simulink model "mat_model"  (R2023a)
settings: Solver=ode4  StartTime=0  StopTime=0.3  FixedStep=1e-7  RelTol=1e-3  EnableMultiTasking=on
undefined symbols (not defined in the file): a_noise, adc_delay_length, ADC_max, adc_sample, b_noise, borehole_max, C_e, C_m, clock_for_random, degrees_shaft_max, delay_ADC, delay_calc_borehole, J_en, J_load, K_degrees2borehole, K_integral, K_noise, K_potentiometer, K_proportional, offset_potentiometer, phi_demanded, q, q_stage, R_rotor, STEP_INTEGRAL, T_rotor, theta_max, U_en_supply, U_ref, width_window
libraries: eePwmGenerator x1
settings Model: SimulationMode=accelerator  Creator=Admin  LastModifiedBy=Director
settings SolverCC: NumberNewtonIterations=4  AlgebraicLoopSolver=TrustRegion  AutoInsertRateTranBlk=on
settings DataIOCC: LimitDataPoints=on  SaveFormat=Array  SignalLoggingSaveFormat=ModelDataLogs  SaveOutput=off  ReturnWorkspaceOutputs=off
settings OptimizationCC: ExpressionDepthLimit=2147483647  LifeSpan=inf  SimCompilerOptimization=on
settings DebuggingCC: UnderspecifiedInitializationDetection=Classic  MergeDetectMultiDrivingBlocksExec=none  SolverPrmCheckMsg=warning  FcnCallInpInsideContextMsg=warning  UnconnectedInputMsg=warning  UnconnectedOutputMsg=warning  UnconnectedLineMsg=warning  StateNameClashWarn=warning  SFUnexpectedBacktrackingDiag=warning  SFNoUnconditionalDefaultTransitionDiag=warning  SFExecutionAtInitializationDiag=none  ArithmeticOperatorsInVariantConditions=warning
settings HardwareCC: ProdBitPerLong=64  ProdLargestAtomicFloat=None  ProdHWDeviceType=AMD->Athlon 64
settings ModelReferenceCC: EnableRefExpFcnMdlSchedulingChecks=on  PropagateSignalLabelsOutOfModel=off
settings SFSimCC: SimUseLocalCustomCode=off  CustomCodeUndefinedFunction=UseInterfaceOnly
settings RTWCC: RTWUseLocalCustomCode=off
settings CodeAppCC: StateflowObjectComments=on
settings GRTTargetCC: TargetLangStandard=C89/C90 (ANSI)  CombineOutputUpdateFcns=off  GRTInterface=on
settings ConfigComp: CovMetricSettings=dw  CovSaveCumulativeToWorkspaceVar=on  CovSaveSingleToWorkspaceVar=on  CovExternalEMLEnable=off
settings SimscapeCC: SimscapeNormalizeSystem=off
settings ConfigurationSet: Description=SimMechanics 2G

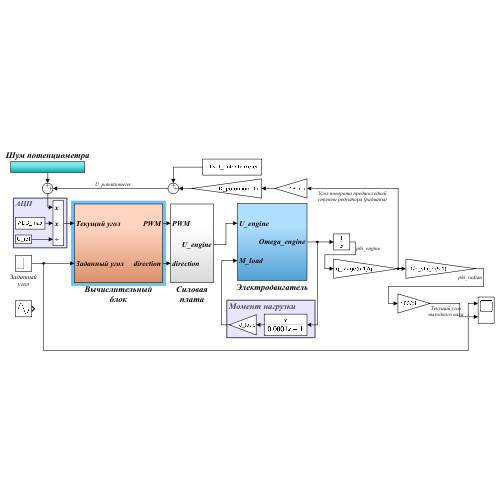
[thumbnail: Simulink's stored preview of the top-level diagram]
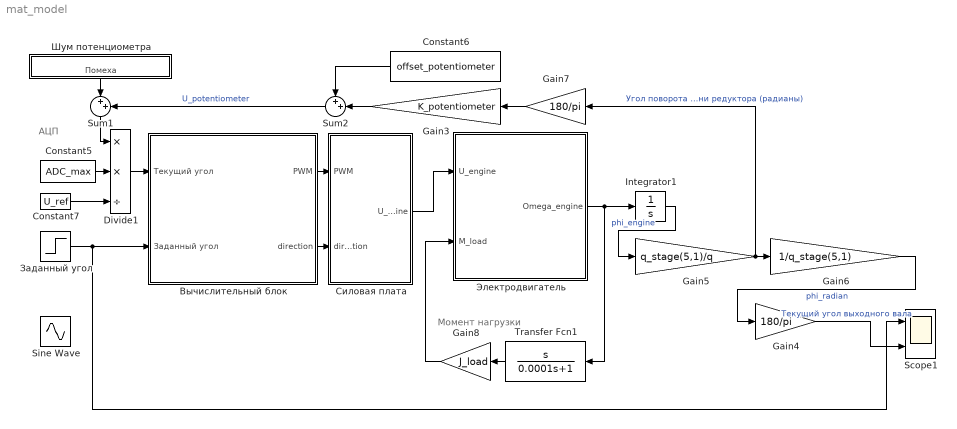
== system mat_model ==
  note: Момент нагрузки
  note: АЦП
  Constant5 : Constant  Value=ADC_max
  Constant6 : Constant  Value=offset_potentiometer
  Constant7 : Constant  Value=U_ref
  Divide1 : Product  Inputs=**/
  Gain3 : Gain  Gain=K_potentiometer
  Gain4 : Gain  Gain=180/pi
  Gain5 : Gain  Gain=q_stage(5,1)/q
  Gain6 : Gain  Gain=1/q_stage(5,1)
  Gain7 : Gain  Gain=180/pi
  Gain8 : Gain  Gain=J_load
  Integrator1 : Integrator
  Scope1 : Scope  NumInputPorts=2
  Sine Wave : Sin  Amplitude=phi_demanded  Frequency=2 * pi * 28.0  SampleTime=0
  Sum1 : Sum  Inputs=|++
  Sum2 : Sum  Inputs=++|
  Transfer Fcn1 : TransferFcn  Numerator=[1 0]  Denominator=[0.0001 1]
  Вычислительный блок : Subsystem
  Заданный угол : Step  Time=0  After=phi_demanded  SampleTime=0
  Силовая плата : Subsystem
  Шум потенциометра : Subsystem
  Электродвигатель : Subsystem
  wires:
  Constant6/1 -> Sum2/1
  Divide1/1 -> Вычислительный блок/1(Текущий угол)
  Gain6/1 -> Gain4/1  "phi_radian"
  Transfer Fcn1/1 -> Gain8/1
  Constant7/1 -> Divide1/3
  Sum1/1 -> Divide1/1
  Gain7/1 -> Gain3/1
  Gain8/1 -> Электродвигатель/2(M_load)
  Integrator1/1 -> Gain5/1  "phi_engine"
  Gain5/1 -> Gain6/1, Gain7/1  "Угол поворота предпоследней ступени редуктора (радианы)"
  Электродвигатель/1(Omega_engine) -> Transfer Fcn1/1, Integrator1/1
  Sum2/1 -> Sum1/2  "U_potentiometer"
  Gain4/1 -> Scope1/2  "Текущий угол выходного вала"
  Constant5/1 -> Divide1/2
  Gain3/1 -> Sum2/2
  Вычислительный блок/1(PWM) -> Силовая плата/1(PWM)
  Вычислительный блок/2(direction) -> Силовая плата/2(direction)
  Силовая плата/1(U_engine) -> Электродвигатель/1(U_engine)
  Заданный угол/1 -> Scope1/1, Вычислительный блок/2(Заданный угол)
  Шум потенциометра/1(Помеха) -> Sum1/1

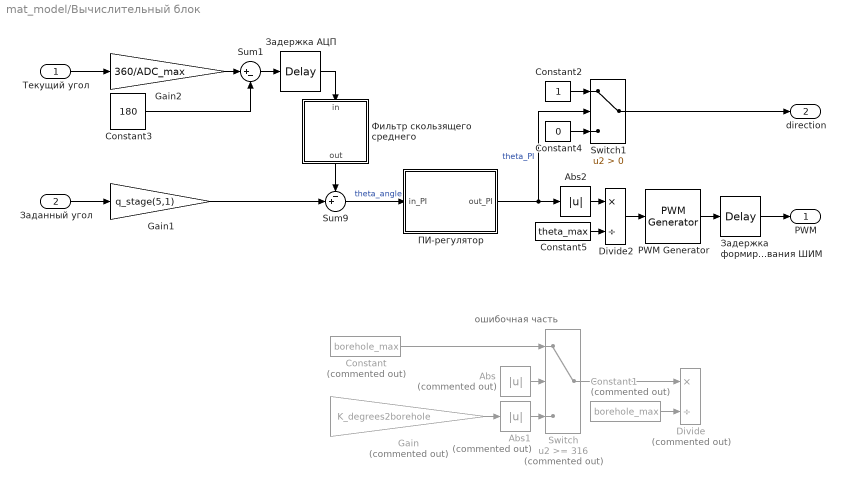
== system mat_model/Вычислительный блок ==
  note: ошибочная часть
  Текущий угол : Inport
  Заданный угол : Inport  Port=2
  Abs : Abs  Commented=on  SaturateOnIntegerOverflow=off
  Abs1 : Abs  Commented=on  SaturateOnIntegerOverflow=off
  Abs2 : Abs  SaturateOnIntegerOverflow=off
  Constant : Constant  Commented=on  Value=borehole_max
  Constant1 : Constant  Commented=on  Value=borehole_max
  Constant2 : Constant
  Constant3 : Constant  Value=180
  Constant4 : Constant  Value=0
  Constant5 : Constant  Value=theta_max
  Divide : Product  Commented=on  Inputs=*/
  Divide2 : Product  Inputs=*/
  Gain : Gain  Commented=on  Gain=K_degrees2borehole
  Gain1 : Gain  Gain=q_stage(5,1)
  Gain2 : Gain  Gain=360/ADC_max
  PWM Generator : eePwmGenerator/PWM Generator  CarrCount=Up  Tper=0.00005  Tdelay=0  Ts=1e-7
  Sum1 : Sum  Inputs=|+-
  Sum9 : Sum  Inputs=-+|
  Switch : Switch  Commented=on  Threshold=316  SaturateOnIntegerOverflow=off  InputSameDT=off
  Switch1 : Switch  Criteria=u2 > Threshold  SaturateOnIntegerOverflow=off  InputSameDT=off
  Задержка формирования ШИМ : TransportDelay  DelayTime=delay_calc_borehole
  Задержка АЦП : TransportDelay  DelayTime=delay_ADC - 0.276*1e-5
  ПИ-регулятор : Subsystem
  Фильтр скользящего среднего : Subsystem
  PWM : Outport
  direction : Outport  Port=2
  wires:
  Sum9/1 -> ПИ-регулятор/1(in_PI)  "theta_angle"
  Задержка формирования ШИМ/1 -> PWM/1
  Constant3/1 -> Sum1/2
  Sum1/1 -> Задержка АЦП/1
  Текущий угол/1 -> Gain2/1
  Gain2/1 -> Sum1/1
  Задержка АЦП/1 -> Фильтр скользящего среднего/1(in)
  Фильтр скользящего среднего/1(out) -> Sum9/1
  Заданный угол/1 -> Gain1/1
  Gain1/1 -> Sum9/2
  Constant/1 -> Switch/1
  Gain/1 -> Abs1/1
  Switch/1 -> Divide/1
  Constant1/1 -> Divide/2
  PWM Generator/1 -> Задержка формирования ШИМ/1
  Constant2/1 -> Switch1/1
  Constant4/1 -> Switch1/3
  Abs/1 -> Switch/2
  Abs1/1 -> Switch/3
  Switch1/1 -> direction/1
  ПИ-регулятор/1(out_PI) -> Switch1/2, Abs2/1  "theta_PI"
  Abs2/1 -> Divide2/1
  Constant5/1 -> Divide2/2
  Divide2/1 -> PWM Generator/1

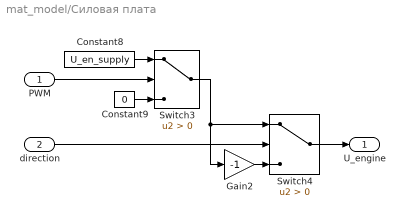
== system mat_model/Силовая плата ==
  PWM : Inport
  direction : Inport  Port=2
  Constant8 : Constant  Value=U_en_supply
  Constant9 : Constant  Value=0
  Gain2 : Gain  Gain=-1
  Switch3 : Switch  Criteria=u2 > Threshold  SaturateOnIntegerOverflow=off  InputSameDT=off
  Switch4 : Switch  Criteria=u2 > Threshold  SaturateOnIntegerOverflow=off  InputSameDT=off
  U_engine : Outport
  wires:
  Constant9/1 -> Switch3/3
  PWM/1 -> Switch3/2
  Switch4/1 -> U_engine/1
  Constant8/1 -> Switch3/1
  direction/1 -> Switch4/2
  Gain2/1 -> Switch4/3
  Switch3/1 -> Switch4/1, Gain2/1

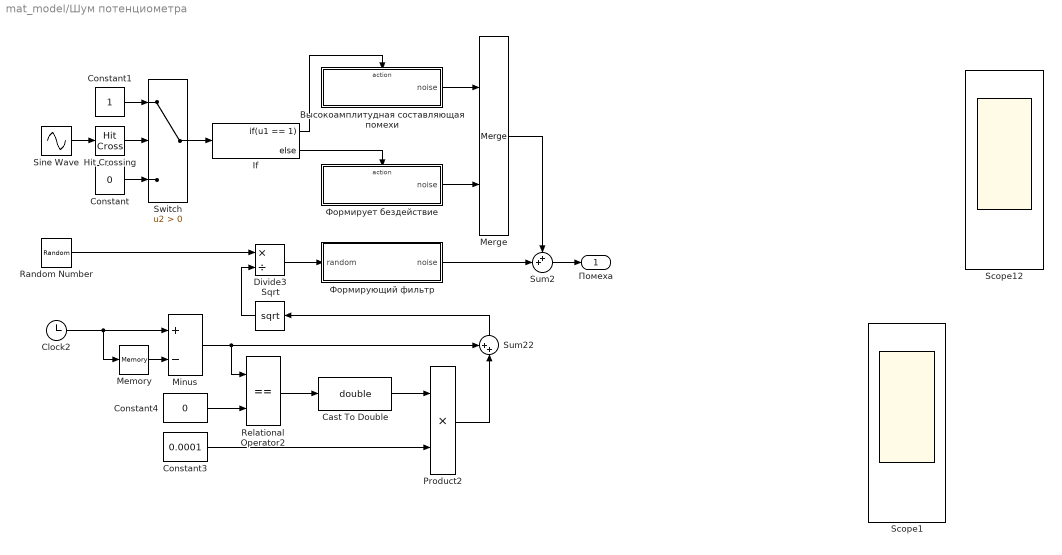
== system mat_model/Шум потенциометра ==
  Cast To Double : DataTypeConversion  OutDataTypeStr=double  SaturateOnIntegerOverflow=off  RndMeth=Floor
  Clock2 : Clock
  Constant : Constant  Value=0
  Constant1 : Constant
  Constant3 : Constant  Value=0.0001
  Constant4 : Constant  Value=0
  Divide3 : Product  Inputs=*/
  Hit Crossing : HitCross  HitCrossingDirection=rising
  If : If  IfExpression=u1 == 1
  Memory : Memory
  Merge : Merge
  Minus : Sum  Inputs=+-
  Product2 : Product
  Random Number : RandomNumber  Seed=clock_for_random(1)  SampleTime=0.00003
  Relational Operator2 : RelationalOperator  Operator===  OutDataTypeStr=boolean  RndMeth=Simplest  InputSameDT=off
  Scope1 : Scope  NumInputPorts=3
  Scope12 : Scope  NumInputPorts=3
  Sine Wave : Sin  Frequency=1350  SampleTime=0
  Sqrt : Sqrt
  Sum2 : Sum  Inputs=++|
  Sum22 : Sum  Inputs=++|
  Switch : Switch  Criteria=u2 > Threshold  SaturateOnIntegerOverflow=off  InputSameDT=off
  Высокоамплитудная составляющая помехи : Subsystem  TreatAsAtomicUnit=on
  Формирует бездействие : Subsystem  TreatAsAtomicUnit=on
  Формирующий фильтр : Subsystem
  Помеха : Outport
  wires:
  Clock2/1 -> Minus/1, Memory/1
  Minus/1 -> Sum22/1, Relational Operator2/1
  Constant3/1 -> Product2/2
  Memory/1 -> Minus/2
  Random Number/1 -> Divide3/1
  Product2/1 -> Sum22/2
  Constant4/1 -> Relational Operator2/2
  Divide3/1 -> Формирующий фильтр/1(random)
  Cast To Double/1 -> Product2/1
  Relational Operator2/1 -> Cast To Double/1
  Sum22/1 -> Sqrt/1
  Sqrt/1 -> Divide3/2
  Формирующий фильтр/1(noise) -> Sum2/2
  Высокоамплитудная составляющая помехи/1(noise) -> Merge/1
  Формирует бездействие/1(noise) -> Merge/2
  Merge/1 -> Sum2/1
  If/1 -> Высокоамплитудная составляющая помехи/Action
  If/2 -> Формирует бездействие/Action
  Constant/1 -> Switch/3
  Constant1/1 -> Switch/1
  Sine Wave/1 -> Hit Crossing/1
  Hit Crossing/1 -> Switch/2
  Switch/1 -> If/1
  Sum2/1 -> Помеха/1

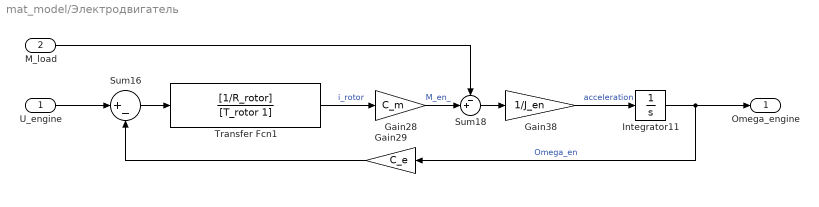
== system mat_model/Электродвигатель ==
  U_engine : Inport
  M_load : Inport  Port=2
  Gain28 : Gain  Gain=C_m
  Gain29 : Gain  Gain=C_e
  Gain38 : Gain  Gain=1/J_en
  Integrator11 : Integrator
  Sum16 : Sum  Inputs=|+-
  Sum18 : Sum  Inputs=-+|
  Transfer Fcn1 : TransferFcn  Numerator=[1/R_rotor]  Denominator=[T_rotor 1]
  Omega_engine : Outport
  wires:
  Integrator11/1 -> Omega_engine/1, Gain29/1  "Omega_en"
  Gain28/1 -> Sum18/2  "M_en_"
  Sum16/1 -> Transfer Fcn1/1
  Gain38/1 -> Integrator11/1  "acceleration"
  Transfer Fcn1/1 -> Gain28/1  "i_rotor"
  Sum18/1 -> Gain38/1
  M_load/1 -> Sum18/1
  U_engine/1 -> Sum16/1
  Gain29/1 -> Sum16/2

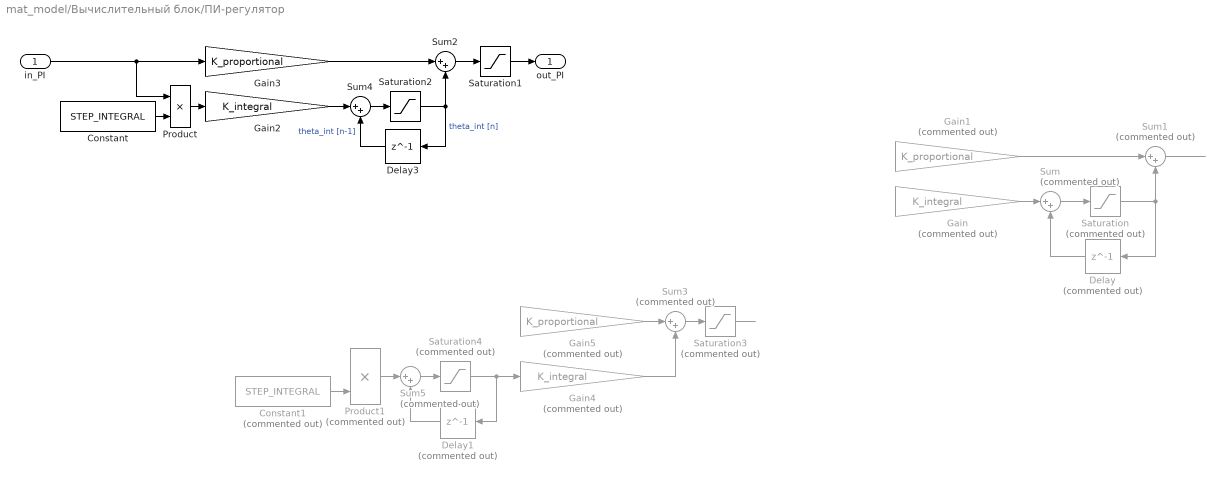
== system mat_model/Вычислительный блок/ПИ-регулятор ==
  in_PI : Inport
  Constant : Constant  Value=STEP_INTEGRAL
  Constant1 : Constant  Commented=on  Value=STEP_INTEGRAL
  Delay : Delay  Commented=on  DelayLength=1  SampleTime=0.0008
  Delay1 : Delay  Commented=on  DelayLength=1  SampleTime=0.000002
  Delay3 : Delay  DelayLength=1  SampleTime=0.000002
  Gain : Gain  Commented=on  Gain=K_integral
  Gain1 : Gain  Commented=on  Gain=K_proportional
  Gain2 : Gain  Gain=K_integral
  Gain3 : Gain  Gain=K_proportional
  Gain4 : Gain  Commented=on  Gain=K_integral
  Gain5 : Gain  Commented=on  Gain=K_proportional
  Product : Product
  Product1 : Product  Commented=on
  Saturation : Saturate  Commented=on
  Saturation1 : Saturate  UpperLimit=316  LowerLimit=-316
  Saturation2 : Saturate
  Saturation3 : Saturate  Commented=on  UpperLimit=316  LowerLimit=-316
  Saturation4 : Saturate  Commented=on
  Sum{,1,3,5} (4 alike) : Sum  Commented=on  Inputs=|++
  Sum2 : Sum  Inputs=|++
  Sum4 : Sum  Inputs=|++
  out_PI : Outport
  wires:
  Constant/1 -> Product/2
  Sum4/1 -> Saturation2/1
  Sum/1 -> Saturation/1
  Gain/1 -> Sum/1
  Saturation/1 -> Delay/1, Sum1/2
  Sum1/1 -> ?
  Delay/1 -> Sum/2
  Gain1/1 -> Sum1/1
  ? -> Gain/1, Gain1/1
  Gain3/1 -> Sum2/1
  in_PI/1 -> Gain3/1, Product/1
  Saturation2/1 -> Sum2/2, Delay3/1  "theta_int [n]"
  Sum2/1 -> Saturation1/1
  Saturation1/1 -> out_PI/1
  Gain4/1 -> Sum3/2
  Sum3/1 -> Saturation3/1
  Saturation3/1 -> ?
  Delay1/1 -> Sum5/2
  Sum5/1 -> Saturation4/1
  Saturation4/1 -> Gain4/1, Delay1/1
  Product1/1 -> Sum5/1
  ? -> Gain5/1, Product1/1
  Gain5/1 -> Sum3/1
  Constant1/1 -> Product1/2
  Product/1 -> Gain2/1
  Gain2/1 -> Sum4/1
  Delay3/1 -> Sum4/2  "theta_int [n-1]"

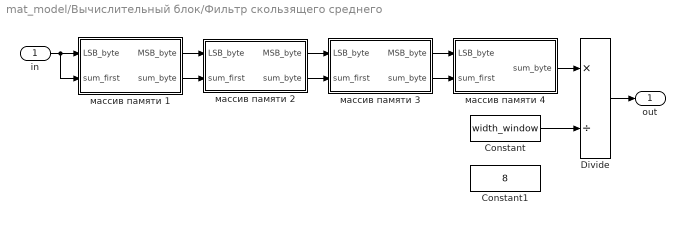
== system mat_model/Вычислительный блок/Фильтр скользящего среднего ==
  in : Inport
  Constant : Constant  Value=width_window
  Constant1 : Constant  Value=8
  Divide : Product  Inputs=*/
  массив памяти 1 : Subsystem
  массив памяти 2 : Subsystem
  массив памяти 3 : Subsystem
  массив памяти 4 : Subsystem
  out : Outport
  wires:
  in/1 -> массив памяти 1/2(sum_first), массив памяти 1/1(LSB_byte)
  Divide/1 -> out/1
  массив памяти 3/1(MSB_byte) -> массив памяти 4/1(LSB_byte)
  массив памяти 3/2(sum_byte) -> массив памяти 4/2(sum_first)
  массив памяти 1/2(sum_byte) -> массив памяти 2/2(sum_first)
  массив памяти 2/1(MSB_byte) -> массив памяти 3/1(LSB_byte)
  массив памяти 2/2(sum_byte) -> массив памяти 3/2(sum_first)
  массив памяти 1/1(MSB_byte) -> массив памяти 2/1(LSB_byte)
  массив памяти 4/1(sum_byte) -> Divide/1
  Constant/1 -> Divide/2

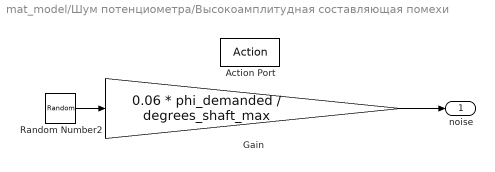
== system mat_model/Шум потенциометра/Высокоамплитудная составляющая помехи ==
  Action Port : ActionPort  ActionPortLabel=if(u1 == 1)
  Gain : Gain  Gain=0.06 * phi_demanded / degrees_shaft_max
  Random Number2 : RandomNumber  Variance=10  Seed=clock_for_random(2)  SampleTime=0
  noise : Outport
  wires:
  Random Number2/1 -> Gain/1
  Gain/1 -> noise/1

== system mat_model/Шум потенциометра/Формирует бездействие ==
  Action Port : ActionPort  ActionPortLabel=else
  Constant : Constant  Value=0
  noise : Outport
  wires:
  Constant/1 -> noise/1

== system mat_model/Шум потенциометра/Формирующий фильтр ==
  random : Inport
  Gain : Gain  Gain=K_noise
  Transfer Fcn : TransferFcn  Denominator=[a_noise b_noise 1]
  noise : Outport
  wires:
  random/1 -> Gain/1
  Gain/1 -> Transfer Fcn/1
  Transfer Fcn/1 -> noise/1

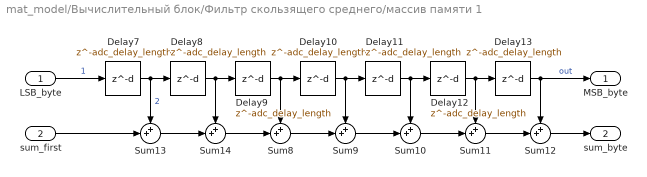
== system mat_model/Вычислительный блок/Фильтр скользящего среднего/массив памяти 1 ==
  LSB_byte : Inport
  sum_first : Inport  Port=2
  Delay{7..13} (7 alike) : Delay  DelayLength=adc_delay_length  SampleTime=adc_sample
  Sum{8..14} (7 alike) : Sum  Inputs=++|
  MSB_byte : Outport
  sum_byte : Outport  Port=2
  wires:
  Delay12/1 -> Sum11/1, Delay13/1
  Delay9/1 -> Delay10/1, Sum8/1
  Sum8/1 -> Sum9/2
  Sum13/1 -> Sum14/2
  Sum9/1 -> Sum10/2
  Sum14/1 -> Sum8/2
  Sum11/1 -> Sum12/2
  Delay11/1 -> Sum10/1, Delay12/1
  Delay10/1 -> Delay11/1, Sum9/1
  Delay7/1 -> Delay8/1, Sum13/1  "2"
  Sum10/1 -> Sum11/2
  Delay8/1 -> Sum14/1, Delay9/1
  Delay13/1 -> MSB_byte/1, Sum12/1  "out"
  Sum12/1 -> sum_byte/1
  LSB_byte/1 -> Delay7/1  "1"
  sum_first/1 -> Sum13/2

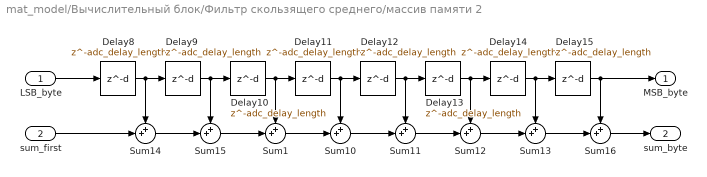
== system mat_model/Вычислительный блок/Фильтр скользящего среднего/массив памяти 2 ==
  LSB_byte : Inport
  sum_first : Inport  Port=2
  Delay{8..15} (8 alike) : Delay  DelayLength=adc_delay_length  SampleTime=adc_sample
  Sum{1,10..16} (8 alike) : Sum  Inputs=++|
  MSB_byte : Outport
  sum_byte : Outport  Port=2
  wires:
  Sum11/1 -> Sum12/2
  Delay9/1 -> Sum15/1, Delay10/1
  Delay8/1 -> Delay9/1, Sum14/1
  Sum15/1 -> Sum1/2
  Delay14/1 -> Delay15/1, Sum13/1
  Sum10/1 -> Sum11/2
  Delay11/1 -> Delay12/1, Sum10/1
  Delay12/1 -> Sum11/1, Delay13/1
  Sum14/1 -> Sum15/2
  Sum12/1 -> Sum13/2
  Delay10/1 -> Delay11/1, Sum1/1
  Sum1/1 -> Sum10/2
  Delay13/1 -> Sum12/1, Delay14/1
  sum_first/1 -> Sum14/2
  Sum13/1 -> Sum16/2
  Delay15/1 -> MSB_byte/1, Sum16/1
  LSB_byte/1 -> Delay8/1
  Sum16/1 -> sum_byte/1

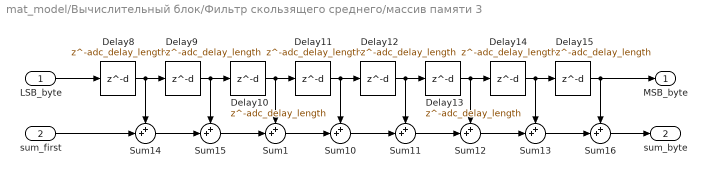
== system mat_model/Вычислительный блок/Фильтр скользящего среднего/массив памяти 3 ==
  LSB_byte : Inport
  sum_first : Inport  Port=2
  Delay{8..15} (8 alike) : Delay  DelayLength=adc_delay_length  SampleTime=adc_sample
  Sum{1,10..16} (8 alike) : Sum  Inputs=++|
  MSB_byte : Outport
  sum_byte : Outport  Port=2
  wires:
  sum_first/1 -> Sum14/2
  Delay15/1 -> MSB_byte/1, Sum16/1
  Delay12/1 -> Sum11/1, Delay13/1
  Sum14/1 -> Sum15/2
  Sum1/1 -> Sum10/2
  Delay13/1 -> Sum12/1, Delay14/1
  Sum13/1 -> Sum16/2
  Delay11/1 -> Delay12/1, Sum10/1
  Delay10/1 -> Delay11/1, Sum1/1
  Delay9/1 -> Sum15/1, Delay10/1
  Delay8/1 -> Delay9/1, Sum14/1
  Sum12/1 -> Sum13/2
  Delay14/1 -> Delay15/1, Sum13/1
  Sum10/1 -> Sum11/2
  Sum11/1 -> Sum12/2
  Sum15/1 -> Sum1/2
  Sum16/1 -> sum_byte/1
  LSB_byte/1 -> Delay8/1

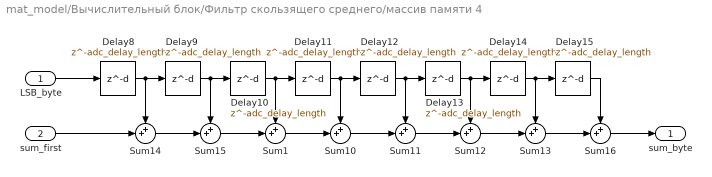
== system mat_model/Вычислительный блок/Фильтр скользящего среднего/массив памяти 4 ==
  LSB_byte : Inport
  sum_first : Inport  Port=2
  Delay{8..14} (7 alike) : Delay  DelayLength=adc_delay_length  SampleTime=adc_sample
  Delay15 : Delay  DelayLength=adc_delay_length
  Sum{1,10..16} (8 alike) : Sum  Inputs=++|
  sum_byte : Outport
  wires:
  Sum1/1 -> Sum10/2
  Delay13/1 -> Sum12/1, Delay14/1
  Delay10/1 -> Delay11/1, Sum1/1
  Sum14/1 -> Sum15/2
  Delay12/1 -> Sum11/1, Delay13/1
  Delay11/1 -> Delay12/1, Sum10/1
  Sum15/1 -> Sum1/2
  Delay14/1 -> Delay15/1, Sum13/1
  Sum12/1 -> Sum13/2
  Delay8/1 -> Delay9/1, Sum14/1
  Delay9/1 -> Sum15/1, Delay10/1
  sum_first/1 -> Sum14/2
  Sum10/1 -> Sum11/2
  Sum13/1 -> Sum16/2
  Delay15/1 -> Sum16/1
  Sum11/1 -> Sum12/2
  Sum16/1 -> sum_byte/1
  LSB_byte/1 -> Delay8/1
